simulink model "AXI_QPSK_Rx"  (R2017b)
settings: Solver=VariableStepAuto  StartTime=0.0  StopTime=2500/Rb  RelTol=1e-3
PreLoadFcn:
  | design_filters_rx;      % run script to generate filter designs.
  | 
  | Rb = 1000;   % 1kbit / s
  | 
  | Rsym = Rb/2;   % 2 bits per symbol
  | 
  | Rsymbol = Rb/2;
  | 
  | OSR = 32;
  | 
  | f_error = 120;
  | 
  | fc = 100e3;
values from neighbouring files (symbols this model uses):
  CIC_fine_Rx = 2^(-(CIC_right_shift_i-CIC_shift_Rx))    [design_filters_rx.m]
  fCIC = fCICcomp * R_CIC    (= 25600000)    [design_filters_rx.m]
  R_CIC = 3200    [design_filters_rx.m]
  R_CICcomp = 2    [design_filters_rx.m]
  R_HB = 2    [design_filters_rx.m]
  R_RRC = 4    [design_filters_rx.m]
undefined symbols (not defined in the file or in its folder): AXI4, designMultirateFIR, Lite
libraries: xbsIndex_r4 x539, dspmlti4 x12, dsparch4 x2, dspsrcs4 x2, commrandsrc2 x1, commdigbbndpm3 x1
(part 1 of 5)
CloseFcn:
  | clear
settings Model: Creator=nas07122  LastModifiedBy=jng
settings CodeAppCC: StateflowObjectComments=on

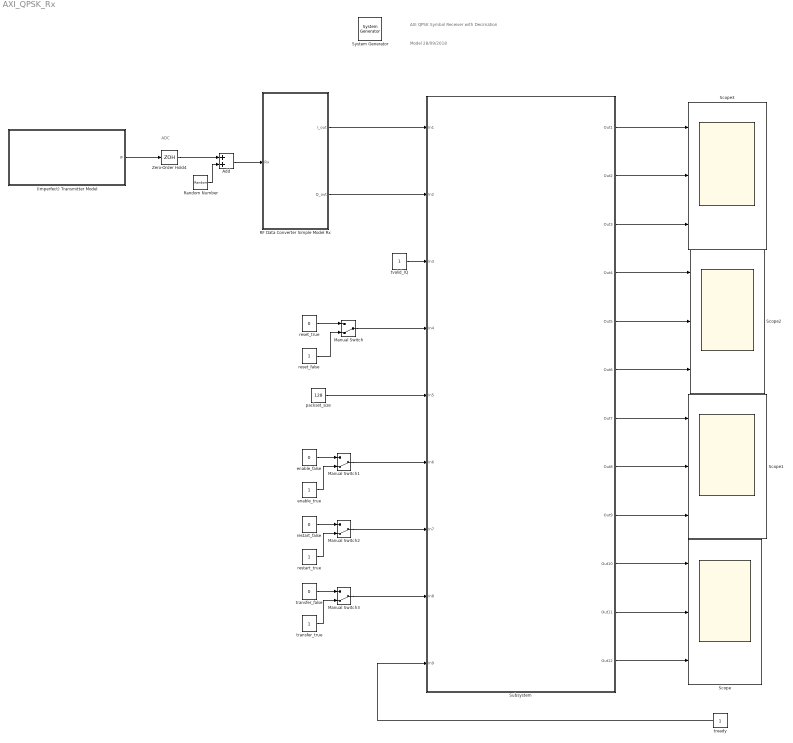
== system AXI_QPSK_Rx ==
  note: ADC
  note: AXI QPSK Symbol Receiver with Decimation
  note: Model 28/09/2018
  " System Generator" : xbsIndex_r4/ System Generator  Tag=genX  xilinxfamily=zynquplusRFSOC  part=xczu28dr  speed=-2-e  package=ffvg1517  synthesis_tool=Vivado  clock_wrapper=Clock Enables  directory=../../iprepo/zcu111/rx  proj_type=Vivado  Synth_file=Vivado Synthesis Defaults  Impl_file=Vivado Implementation Defaults  testbench=off  simulink_period=1/(0.5*Rb*R_RRC*R_HB*R_CICcomp*R_CIC)  sysclk_period=10  dcm_input_clock_period=10  incr_netlist=off  trim_vbits=Everywhere in SubSystem  dbl_ovrd=According to Block Masks  core_generation=According to Block Masks  run_coregen=off  deprecated_control=off  eval_field=0  block_type=sysgen
  (Imperfect) Transmitter Model : Subsystem  mask(Model of a QPSK Transmitter with Timing and Frequency Offsets){T_error=5, F_error=f_error, fc=fc}
      mask prompts: T_error "Timing Error (ppm)"; F_error "Frequency Error (Hz)"; fc "IF Carrier Frequency (Hz)"
      mask help:
      | Enter the timing and frequency offsets that apply to the received signal.
      |
      | Both of these can be negative or positive values. Negative means that the timing / frequency of the transmitter is lower than expected.
      mask init:
      | T_Offset = 1+(T_error/1e6);
      | F_Offset = F_error;
  Add : Sum
  Manual Switch{,1..3} (4 alike) : ManualSwitch  CurrentSetting=0
  RF Data Converter Simple Model Rx : Subsystem
  Random Number : RandomNumber  Variance=0.05  SampleTime=1/(0.5*R_RRC*R_HB*R_CICcomp*R_CIC*8*Rb)
  Scope{,1..3} (4 alike) : Scope  NumInputPorts=3
  Subsystem : Subsystem
  Zero-Order Hold4 : ZeroOrderHold  SampleTime=1/(0.5*R_RRC*R_HB*R_CICcomp*R_CIC*8*Rb)
  enable_false : Constant  Value=0  VectorParams1D=off  OutDataTypeStr=boolean  SampleTime=-1
  enable_true : Constant  VectorParams1D=off  OutDataTypeStr=boolean  SampleTime=-1
  packset_size : Constant  Value=128  SampleTime=-1
  reset_false : Constant  VectorParams1D=off  OutDataTypeStr=boolean  SampleTime=-1
  reset_true : Constant  Value=0  VectorParams1D=off  OutDataTypeStr=boolean  SampleTime=-1
  restart_false : Constant  Value=0  VectorParams1D=off  OutDataTypeStr=boolean  SampleTime=-1
  restart_true : Constant  VectorParams1D=off  OutDataTypeStr=boolean  SampleTime=-1
  transfer_false : Constant  Value=0  VectorParams1D=off  OutDataTypeStr=boolean  SampleTime=-1
  transfer_true : Constant  VectorParams1D=off  OutDataTypeStr=boolean  SampleTime=-1
  tready : Constant  SampleTime=-1
  tvalid_IQ : Constant  VectorParams1D=off  OutDataTypeStr=boolean  SampleTime=-1
  wires:
  Add/1 -> RF Data Converter Simple Model Rx/1(Rx)
  Zero-Order Hold4/1 -> Add/1
  Random Number/1 -> Add/2
  (Imperfect) Transmitter Model/1(IF) -> Zero-Order Hold4/1
  enable_true/1 -> Manual Switch1/2
  transfer_false/1 -> Manual Switch3/1
  reset_true/1 -> Manual Switch/1
  transfer_true/1 -> Manual Switch3/2
  restart_false/1 -> Manual Switch2/1
  enable_false/1 -> Manual Switch1/1
  restart_true/1 -> Manual Switch2/2
  reset_false/1 -> Manual Switch/2
  RF Data Converter Simple Model Rx/1(I_out) -> Subsystem/1(In1)
  RF Data Converter Simple Model Rx/2(Q_out) -> Subsystem/2(In2)
  tvalid_IQ/1 -> Subsystem/3(In3)
  Manual Switch/1 -> Subsystem/4(In4)
  packset_size/1 -> Subsystem/5(In5)
  Manual Switch1/1 -> Subsystem/6(In6)
  Manual Switch2/1 -> Subsystem/7(In7)
  Manual Switch3/1 -> Subsystem/8(In8)
  tready/1 -> Subsystem/9(In9)
  Subsystem/1(Out1) -> Scope3/1
  Subsystem/2(Out2) -> Scope3/2
  Subsystem/3(Out3) -> Scope3/3
  Subsystem/4(Out4) -> Scope2/1
  Subsystem/5(Out5) -> Scope2/2
  Subsystem/6(Out6) -> Scope2/3
  Subsystem/7(Out7) -> Scope1/1
  Subsystem/8(Out8) -> Scope1/2
  Subsystem/9(Out9) -> Scope1/3
  Subsystem/10(Out10) -> Scope/1
  Subsystem/11(Out11) -> Scope/2
  Subsystem/12(Out12) -> Scope/3

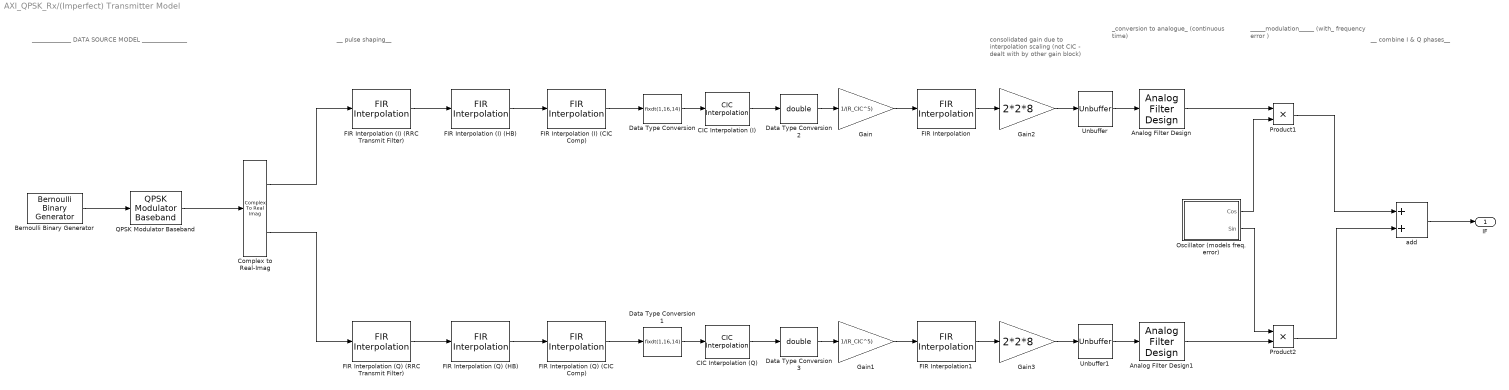
== system AXI_QPSK_Rx/(Imperfect) Transmitter Model ==
  note: consolidated gain
      | due to interpolation scaling
      | (not CIC - dealt with by other
      | gain block)
  note: _____________ DATA SOURCE MODEL _______________
  note: _conversion to analogue_
      | (continuous time)
  note: __ pulse shaping__
  note: _____modulation_____
      | (with_ frequency error )
  note: __ combine I & Q phases__
  Analog Filter Design : dsparch4/Analog Filter Design  method=Butterworth  filttype=Lowpass  N=8  Wlo=2*pi*Rsymbol*T_Offset  Whi=80  Rp=2  Rs=40
  Analog Filter Design1 : dsparch4/Analog Filter Design  method=Butterworth  filttype=Lowpass  N=8  Wlo=2*pi*Rsymbol*T_Offset  Whi=80  Rp=2  Rs=40
  Bernoulli Binary Generator : commrandsrc2/Bernoulli Binary Generator  P=0.5  seed=61  Ts=1/(T_Offset*Rb)  frameBased=on  sampPerFrame=2  orient=off  outDataType=double
  CIC Interpolation (I) : dspmlti4/CIC Interpolation  filtFrom=Dialog  filtobj=CICINTERP  ftype=Interpolator  R=R_CIC  M=1  N=5  filterInternals=Full precision  BPS=[16 16 16 16]  FLPS=0  outputWordLength=32  outputFracLength=0  launchFVT=off  framing=Enforce single-rate processing  InputProcessing=Columns as channels (frame based)  OutputFrames=off
      settings: SourceProductName=DSP System Toolbox  SourceProductBaseCode=DS
  CIC Interpolation (Q) : dspmlti4/CIC Interpolation  filtFrom=Dialog  filtobj=CICINTERP  ftype=Interpolator  R=R_CIC  M=1  N=5  filterInternals=Full precision  BPS=[16 16 16 16]  FLPS=0  outputWordLength=32  outputFracLength=0  launchFVT=off  framing=Enforce single-rate processing  InputProcessing=Columns as channels (frame based)  OutputFrames=off
      settings: SourceProductName=DSP System Toolbox  SourceProductBaseCode=DS
  Complex to Real-Imag : ComplexToRealImag
  Data Type Conversion : DataTypeConversion  OutDataTypeStr=fixdt(1,16,14)
  Data Type Conversion1 : DataTypeConversion  OutDataTypeStr=fixdt(1,16,14)
  Data Type Conversion2 : DataTypeConversion  OutDataTypeStr=double
  Data Type Conversion3 : DataTypeConversion  OutDataTypeStr=double
  FIR Interpolation : dspmlti4/FIR Interpolation  FilterSource=Auto  h=designMultirateFIR(3,1)  L=8  FilterObject=FINTERP  InputProcessing=Columns as channels (frame based)  framing=Allow multirate processing  outputBufInitCond=0  roundingMode=Floor  overflowMode=off  firstCoeffDataTypeStr=Inherit: Same word length as input  firstCoeffMin=[]  firstCoeffMax=[]  firstCoeffLastDataTypeStr=Inherit: Same word length as input  outputDataTypeStr=Inherit: Same as accumulator  outputMin=[]  outputMax=[]  outputLastDataTypeStr=Inherit: Same as accumulator
      settings: SourceProductName=DSP System Toolbox
  FIR Interpolation1 : dspmlti4/FIR Interpolation  FilterSource=Auto  h=designMultirateFIR(3,1)  L=8  FilterObject=FINTERP  InputProcessing=Columns as channels (frame based)  framing=Allow multirate processing  outputBufInitCond=0  roundingMode=Floor  overflowMode=off  firstCoeffDataTypeStr=Inherit: Same word length as input  firstCoeffMin=[]  firstCoeffMax=[]  firstCoeffLastDataTypeStr=Inherit: Same word length as input  outputDataTypeStr=Inherit: Same as accumulator  outputMin=[]  outputMax=[]  outputLastDataTypeStr=Inherit: Same as accumulator
      settings: SourceProductName=DSP System Toolbox
  FIR Interpolation (I) (CIC Comp) : dspmlti4/FIR Interpolation  FilterSource=Dialog parameters  h=WComp.Numerator  L=R_CICcomp  FilterObject=FINTERP  InputProcessing=Columns as channels (frame based)  framing=Allow multirate processing  outputBufInitCond=0  roundingMode=Floor  overflowMode=off  firstCoeffDataTypeStr=Inherit: Same word length as input  firstCoeffMin=[]  firstCoeffMax=[]  firstCoeffLastDataTypeStr=Inherit: Same word length as input  outputDataTypeStr=Inherit: Same as accumulator  outputMin=[]  outputMax=[]  outputLastDataTypeStr=Inherit: Same as accumulator
      settings: SourceProductName=DSP System Toolbox
  FIR Interpolation (I) (HB) : dspmlti4/FIR Interpolation  FilterSource=Dialog parameters  h=HB.Numerator  L=2  FilterObject=FINTERP  InputProcessing=Columns as channels (frame based)  framing=Allow multirate processing  outputBufInitCond=0  roundingMode=Floor  overflowMode=off  firstCoeffDataTypeStr=Inherit: Same word length as input  firstCoeffMin=[]  firstCoeffMax=[]  firstCoeffLastDataTypeStr=Inherit: Same word length as input  outputDataTypeStr=Inherit: Same as accumulator  outputMin=[]  outputMax=[]  outputLastDataTypeStr=Inherit: Same as accumulator
      settings: SourceProductName=DSP System Toolbox
  FIR Interpolation (I) (RRC Transmit Filter) : dspmlti4/FIR Interpolation  FilterSource=Dialog parameters  h=WRRC.Numerator  L=R_RRC  FilterObject=FINTERP  InputProcessing=Columns as channels (frame based)  framing=Allow multirate processing  outputBufInitCond=0  roundingMode=Floor  overflowMode=off  firstCoeffDataTypeStr=Inherit: Same word length as input  firstCoeffMin=[]  firstCoeffMax=[]  firstCoeffLastDataTypeStr=Inherit: Same word length as input  outputDataTypeStr=Inherit: Same as accumulator  outputMin=[]  outputMax=[]  outputLastDataTypeStr=Inherit: Same as accumulator
      settings: SourceProductName=DSP System Toolbox
  FIR Interpolation (Q) (CIC Comp) : dspmlti4/FIR Interpolation  FilterSource=Dialog parameters  h=WComp.Numerator  L=R_CICcomp  FilterObject=FINTERP  InputProcessing=Columns as channels (frame based)  framing=Allow multirate processing  outputBufInitCond=0  roundingMode=Floor  overflowMode=off  firstCoeffDataTypeStr=Inherit: Same word length as input  firstCoeffMin=[]  firstCoeffMax=[]  firstCoeffLastDataTypeStr=Inherit: Same word length as input  outputDataTypeStr=Inherit: Same as accumulator  outputMin=[]  outputMax=[]  outputLastDataTypeStr=Inherit: Same as accumulator
      settings: SourceProductName=DSP System Toolbox
  FIR Interpolation (Q) (HB) : dspmlti4/FIR Interpolation  FilterSource=Dialog parameters  h=HB.Numerator  L=2  FilterObject=FINTERP  InputProcessing=Columns as channels (frame based)  framing=Allow multirate processing  outputBufInitCond=0  roundingMode=Floor  overflowMode=off  firstCoeffDataTypeStr=Inherit: Same word length as input  firstCoeffMin=[]  firstCoeffMax=[]  firstCoeffLastDataTypeStr=Inherit: Same word length as input  outputDataTypeStr=Inherit: Same as accumulator  outputMin=[]  outputMax=[]  outputLastDataTypeStr=Inherit: Same as accumulator
      settings: SourceProductName=DSP System Toolbox
  FIR Interpolation (Q) (RRC Transmit Filter) : dspmlti4/FIR Interpolation  FilterSource=Dialog parameters  h=WRRC.Numerator  L=R_RRC  FilterObject=FINTERP  InputProcessing=Columns as channels (frame based)  framing=Allow multirate processing  outputBufInitCond=0  roundingMode=Floor  overflowMode=off  firstCoeffDataTypeStr=Inherit: Same word length as input  firstCoeffMin=[]  firstCoeffMax=[]  firstCoeffLastDataTypeStr=Inherit: Same word length as input  outputDataTypeStr=Inherit: Same as accumulator  outputMin=[]  outputMax=[]  outputLastDataTypeStr=Inherit: Same as accumulator
      settings: SourceProductName=DSP System Toolbox
  Gain : Gain  Gain=1/(R_CIC^5)
  Gain1 : Gain  Gain=1/(R_CIC^5)
  Gain2 : Gain  Gain=2*2*8
  Gain3 : Gain  Gain=2*2*8
  Oscillator (models freq. error) : Subsystem
  Product1 : Product
  Product2 : Product
  QPSK Modulator Baseband : commdigbbndpm3/QPSK Modulator Baseband  InType=Bit  Enc=Gray  Ph=pi/4  outDtype=double  outWordLen=16  outUDDataType=sfix(16)  outFracLenMode=Best precision  outFracLen=15  outDataTypeStr=double  outLastDataTypeStr=double
  Unbuffer : Unbuffer
  Unbuffer1 : Unbuffer
  add : Sum
  IF : Outport
  wires:
  FIR Interpolation (Q) (RRC Transmit Filter)/1 -> FIR Interpolation (Q) (HB)/1
  Complex to Real-Imag/2 -> FIR Interpolation (Q) (RRC Transmit Filter)/1
  Complex to Real-Imag/1 -> FIR Interpolation (I) (RRC Transmit Filter)/1
  Bernoulli Binary Generator/1 -> QPSK Modulator Baseband/1
  FIR Interpolation (I) (RRC Transmit Filter)/1 -> FIR Interpolation (I) (HB)/1
  Product1/1 -> add/1
  Analog Filter Design/1 -> Product1/1
  Analog Filter Design1/1 -> Product2/2
  Product2/1 -> add/2
  add/1 -> IF/1
  Oscillator (models freq. error)/1(Cos) -> Product1/2
  Oscillator (models freq. error)/2(Sin) -> Product2/1
  QPSK Modulator Baseband/1 -> Complex to Real-Imag/1
  Unbuffer/1 -> Analog Filter Design/1
  Unbuffer1/1 -> Analog Filter Design1/1
  FIR Interpolation (I) (HB)/1 -> FIR Interpolation (I) (CIC Comp)/1
  FIR Interpolation (Q) (HB)/1 -> FIR Interpolation (Q) (CIC Comp)/1
  FIR Interpolation (I) (CIC Comp)/1 -> Data Type Conversion/1
  FIR Interpolation (Q) (CIC Comp)/1 -> Data Type Conversion1/1
  CIC Interpolation (I)/1 -> Data Type Conversion2/1
  CIC Interpolation (Q)/1 -> Data Type Conversion3/1
  FIR Interpolation/1 -> Gain2/1
  FIR Interpolation1/1 -> Gain3/1
  Data Type Conversion/1 -> CIC Interpolation (I)/1
  Data Type Conversion1/1 -> CIC Interpolation (Q)/1
  Data Type Conversion2/1 -> Gain/1
  Data Type Conversion3/1 -> Gain1/1
  Gain/1 -> FIR Interpolation/1
  Gain1/1 -> FIR Interpolation1/1
  Gain2/1 -> Unbuffer/1
  Gain3/1 -> Unbuffer1/1

== system AXI_QPSK_Rx/RF Data Converter Simple Model Rx ==
  Rx : Inport
  Cosine Wave : dspsrcs4/Sine Wave  Amplitude=1  Frequency=fc  Phase=pi/2  SampleMode=Discrete  OutComplex=Real  CompMethod=Trigonometric fcn  TableSize=Speed  SampleTime=1/(0.5*R_RRC*R_HB*R_CICcomp*R_CIC*8*Rb)  SamplesPerFrame=1  ResetState=Restart at time zero  OutputFrames=off  dataType=double  wordLen=16  udDataType=sfix(16)  fracBitsMode=Best precision  numFracBits=15  OutDataTypeStr=double  LastOutDataTypeStr=double
  FIR Decimation : dspmlti4/FIR Decimation  FilterSource=Auto  h=designMultirateFIR(1,2)  D=8  filtStruct=Direct form  FilterObject=FDECIM  framing=Enforce single-rate processing  inputOffset=0  outputBufInitCond=0  roundingMode=Floor  overflowMode=off  firstCoeffDataTypeStr=Inherit: Same word length as input  firstCoeffMin=[]  firstCoeffMax=[]  firstCoeffLastDataTypeStr=Inherit: Same word length as input  outputDataTypeStr=Inherit: Same as accumulator  outputMin=[]  outputMax=[]  outputLastDataTypeStr=Inherit: Same as accumulator
  FIR Decimation1 : dspmlti4/FIR Decimation  FilterSource=Auto  h=designMultirateFIR(1,2)  D=8  filtStruct=Direct form  FilterObject=FDECIM  framing=Enforce single-rate processing  inputOffset=0  outputBufInitCond=0  roundingMode=Floor  overflowMode=off  firstCoeffDataTypeStr=Inherit: Same word length as input  firstCoeffMin=[]  firstCoeffMax=[]  firstCoeffLastDataTypeStr=Inherit: Same word length as input  outputDataTypeStr=Inherit: Same as accumulator  outputMin=[]  outputMax=[]  outputLastDataTypeStr=Inherit: Same as accumulator
  Product : Product
  Product1 : Product
  Sine Wave : dspsrcs4/Sine Wave  Amplitude=1  Frequency=fc  Phase=pi  SampleMode=Discrete  OutComplex=Real  CompMethod=Trigonometric fcn  TableSize=Speed  SampleTime=1/(0.5*R_RRC*R_HB*R_CICcomp*R_CIC*8*Rb)  SamplesPerFrame=1  ResetState=Restart at time zero  OutputFrames=off  dataType=double  wordLen=16  udDataType=sfix(16)  fracBitsMode=Best precision  numFracBits=15  OutDataTypeStr=double  LastOutDataTypeStr=double
  I_out : Outport
  Q_out : Outport  Port=2
  wires:
  FIR Decimation/1 -> I_out/1
  Rx/1 -> Product1/2, Product/1
  Cosine Wave/1 -> Product/2
  Product/1 -> FIR Decimation/1
  Sine Wave/1 -> Product1/1
  Product1/1 -> FIR Decimation1/1
  FIR Decimation1/1 -> Q_out/1

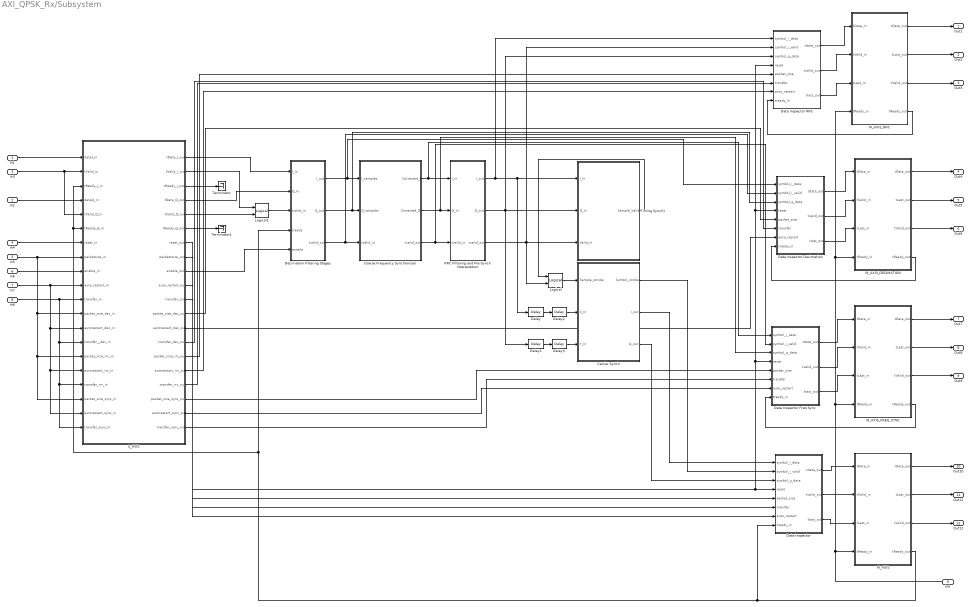
== system AXI_QPSK_Rx/Subsystem ==
  In1 : Inport
  In2 : Inport  Port=2
  In3 : Inport  Port=3
  In4 : Inport  Port=4
  In5 : Inport  Port=5
  In6 : Inport  Port=6
  In7 : Inport  Port=7
  In8 : Inport  Port=8
  In9 : Inport  Port=9
  Carrier Synch : Subsystem  mask(Symbol Timing Synchroniser){Rsymbol=Rsymbol}
      mask prompts: Rsymbol "Symbol rate (Hz)"
      mask init:
      | d = 0.707;                  % damping ratio 
      | 
      | % *** CARRIER synch loop *** (note this operates at symbol rate)
      | 
      | T = 1/Rsymbol;               % sample period
      | Kp = 1;                      % phase detector S-curve is linear
      | Bn = 0.04*Rsymbol;           % bandwidth in Hz
      | Ko = 1;                      % gain of NCO 
      | 
      | % calculate the loop filter coefficients for the carrier synch loop
      | K1 = (4*d*Bn*T)/(Ko*Kp*(d+1/(4*d)));
      | K2 = (4*(Bn*T)^2)/(Ko*Kp*(d+1/4*d)^2);
  Coarse Frequency Synchroniser : Subsystem  mask(Coarse Frequency Synchronisation (QPSK)){f_coarse=(0.5*R_RRC*R_HB*Rb), Nfft=512}
      mask prompts: f_coarse "Sampling frequency"; Nfft "FFT size (must be power of 2)"
      mask help: This coarse synchronisation block raises the received signal to the power of M = 4 (for QPSK, i.e. the modulation order) and finds the peak in the resulting spectrum, to identify the frequency offset from baseband. A complex exponential at the identified frequency is then generated and used to perform a frequency correction on the received signal.
      mask init:
      | M = 4;      % for QPSK
      | 
      | % set FFT block to size specified in mask.
      | set_param([gcb,'/FFT'],'transform_length',num2str(Nfft));      
      | 
      | % generate lookup table for frequency correction term
      | fcorr_lookup = zeros(1,Nfft);
      | 
      | n = (0:Nfft-1);
      | fcorr_lookup(1:Nfft/2) = - (n(1:Nfft/2) * (f_coarse/(4*Nfft)));
      | fcorr_lookup((Nfft/2)+1:end) = - ((n((Nfft/2)+1:end) - Nfft) *  (f_coarse/(4*Nfft)));
  Data Inspector : Subsystem
  Data Inspector Decimation : Subsystem
  Data Inspector Freq Sync : Subsystem
  Data Inspector RRC : Subsystem
  Decimation Filtering Stages : Subsystem
  Delay : xbsIndex_r4/Delay  rst=off  infoeditControl=Selection of Reset will increase slice count due to use of real FFs and instead of SRLs  en=off  latency=OSR/2  reg_retiming=off  dbl_ovrd=off  block_type=delay
  Delay1 : xbsIndex_r4/Delay  rst=off  infoeditControl=Selection of Reset will increase slice count due to use of real FFs and instead of SRLs  en=off  latency=OSR/2  reg_retiming=off  dbl_ovrd=off  block_type=delay
  Delay2 : xbsIndex_r4/Delay  rst=off  infoeditControl=Selection of Reset will increase slice count due to use of real FFs and instead of SRLs  en=off  latency=1  reg_retiming=off  dbl_ovrd=off  block_type=delay
  Delay3 : xbsIndex_r4/Delay  rst=off  infoeditControl=Selection of Reset will increase slice count due to use of real FFs and instead of SRLs  en=off  latency=1  reg_retiming=off  dbl_ovrd=off  block_type=delay
  Logical : xbsIndex_r4/Logical  logical_function=AND  inputs=2  en=off  latency=0  precision=Full  arith_type=Unsigned  n_bits=16  bin_pt=0  align_bp=on  dbl_ovrd=off  block_type=logical
  Logical1 : xbsIndex_r4/Logical  logical_function=AND  inputs=2  en=off  latency=0  precision=Full  arith_type=Unsigned  n_bits=16  bin_pt=0  align_bp=on  dbl_ovrd=off  block_type=logical
  M_AXIS : Subsystem
  M_AXIS_DECIMATION : Subsystem
  M_AXIS_FREQ_SYNC : Subsystem
  M_AXIS_RRC : Subsystem
  "RRC Filtering and Pre-Synch Interpolation " : Subsystem
  S_AXIS : Subsystem
  Terminator : Terminator
  Terminator1 : Terminator
  Timing Synch1 : Subsystem  mask(Symbol Timing Synchroniser){Rsymbol=Rsymbol}
      mask prompts: Rsymbol "Symbol rate (Hz)"
      mask init:
      | % *** SYMBOL TIMING synch loop ***
      | 
      | d = 0.707;                  % damping ratio 
      | Ts = 1/Rsymbol;             % symbol period
      | Ks = 3.24;                  % phase detector coefficient
      | BnS = 0.08*Rsymbol;         % bandwidth in Hz
      | Kn   = 1;                   % gain of numerically controlled clock
      | 
      | % calculate loop filter coefficients
      | Ka = (4*d*BnS*Ts)/(Kn*Ks*(d+1/(4*d)));
      | Kb = (4*(BnS*Ts)^2)/(Kn*Ks*(d+1/4*d)^2);
  Out1 : Outport
  Out2 : Outport  Port=2
  Out3 : Outport  Port=3
  Out4 : Outport  Port=4
  Out5 : Outport  Port=5
  Out6 : Outport  Port=6
  Out7 : Outport  Port=7
  Out8 : Outport  Port=8
  Out9 : Outport  Port=9
  Out10 : Outport  Port=10
  Out11 : Outport  Port=11
  Out12 : Outport  Port=12
  wires:
  Coarse Frequency Synchroniser/1(Corrected_I) -> Data Inspector Freq Sync/1(symbol_i_data), "RRC Filtering and Pre-Synch Interpolation "/1(I_in)
  In2/1 -> S_AXIS/4(dataQ_in)
  M_AXIS_FREQ_SYNC/1(tData_out) -> Out7/1
  Data Inspector Freq Sync/2(tvalid_out) -> M_AXIS_FREQ_SYNC/2(tValid_in)
  In5/1 -> S_AXIS/8(packetsize_in), S_AXIS/12(packet_size_dec_in), S_AXIS/15(packet_size_rrc_in), S_AXIS/18(packet_size_sync_in)
  S_AXIS/16(autorestart_rrc_out) -> Data Inspector RRC/7(auto_restart)
  S_AXIS/19(autorestart_sync_out) -> Data Inspector Freq Sync/7(auto_restart)
  S_AXIS/10(auto_restart_out) -> Data Inspector/7(auto_restart)
  S_AXIS/13(autorestart_dec_out) -> Data Inspector Decimation/7(auto_restart)
  S_AXIS/1(tData_I_out) -> Decimation Filtering Stages/1(I_In)
  In9/1 -> M_AXIS/4(tReady_in), M_AXIS_FREQ_SYNC/4(tReady_in), M_AXIS_DECIMATION/4(tReady_in), M_AXIS_RRC/4(tReady_in)
  S_AXIS/6(tReady_Q_out) -> Terminator1/1
  Data Inspector/2(tvalid_out) -> M_AXIS/2(tValid_in)
  M_AXIS_DECIMATION/4(tReady_out) -> Data Inspector Decimation/8(tready_in)
  In6/1 -> S_AXIS/9(enable_in)
  Timing Synch1/1(Sample_Valid) -> Logical/1
  "RRC Filtering and Pre-Synch Interpolation "/3(tvalid_out) -> Data Inspector RRC/2(symbol_i_valid), Timing Synch1/3(Valid_in), Logical/2
  M_AXIS_DECIMATION/2(tLast_out) -> Out5/1
  Delay/1 -> Delay2/1
  Delay1/1 -> Delay3/1
  Logical1/1 -> Decimation Filtering Stages/3(tvalid_in)
  Logical/1 -> Carrier Synch/1(Sample_strobe)
  M_AXIS_FREQ_SYNC/2(tLast_out) -> Out8/1
  Carrier Synch/1(Symbol_strobe) -> Data Inspector/2(symbol_i_valid)
  S_AXIS/2(tValid_I_out) -> Logical1/1
  M_AXIS_RRC/3(tValid_out) -> Out3/1
  M_AXIS_FREQ_SYNC/4(tReady_out) -> Data Inspector Freq Sync/8(tready_in)
  S_AXIS/5(tValid_Q_out) -> Logical1/2
  Carrier Synch/3(Q_out) -> Data Inspector/3(symbol_q_data)
  Decimation Filtering Stages/2(Q_out) -> Data Inspector Decimation/3(symbol_q_data), Coarse Frequency Synchroniser/2(Q_samples)
  In8/1 -> S_AXIS/11(transfer_in), S_AXIS/14(transfer__dec_in), S_AXIS/17(transfer_rrc_in), S_AXIS/20(transfer_sync_in)
  Data Inspector Decimation/3(tlast_out) -> M_AXIS_DECIMATION/3(tLast_in)
  Data Inspector/3(tlast_out) -> M_AXIS/3(tLast_in)
  S_AXIS/4(tData_Q_out) -> Decimation Filtering Stages/2(Q_In)
  Data Inspector RRC/2(tvalid_out) -> M_AXIS_RRC/2(tValid_in)
  S_AXIS/18(packet_size_sync_out) -> Data Inspector Freq Sync/5(packet_size)
  M_AXIS_DECIMATION/3(tValid_out) -> Out6/1
  Data Inspector RRC/1(tdata_out) -> M_AXIS_RRC/1(tData_in)
  In3/1 -> S_AXIS/5(tValid_Q_in), S_AXIS/2(tValid_in)
  Data Inspector Freq Sync/1(tdata_out) -> M_AXIS_FREQ_SYNC/1(tData_in)
  Coarse Frequency Synchroniser/3(tvalid_out) -> Data Inspector Freq Sync/2(symbol_i_valid), "RRC Filtering and Pre-Synch Interpolation "/3(tvalid_in)
  Data Inspector RRC/3(tlast_out) -> M_AXIS_RRC/3(tLast_in)
  Data Inspector Decimation/2(tvalid_out) -> M_AXIS_DECIMATION/2(tValid_in)
  In7/1 -> S_AXIS/19(autorestart_sync_in), S_AXIS/16(autorestart_rrc_in), S_AXIS/13(autorestart_dec_in), S_AXIS/10(auto_restart_in)
  M_AXIS_RRC/4(tReady_out) -> Data Inspector RRC/8(tready_in)
  M_AXIS/3(tValid_out) -> Out12/1
  Data Inspector/1(tdata_out) -> M_AXIS/1(tData_in)
  S_AXIS/8(packsetsize_out) -> Data Inspector/5(packet_size)
  S_AXIS/14(transfer_dec_out) -> Data Inspector Decimation/6(transfer)
  Data Inspector Freq Sync/3(tlast_out) -> M_AXIS_FREQ_SYNC/3(tLast_in)
  S_AXIS/11(transfer_out) -> Data Inspector/6(transfer)
  Delay2/1 -> Carrier Synch/2(X_In)
  Data Inspector Decimation/1(tdata_out) -> M_AXIS_DECIMATION/1(tData_in)
  S_AXIS/15(packet_size_rrc_out) -> Data Inspector RRC/5(packet_size)
  Delay3/1 -> Carrier Synch/3(Y_In)
  M_AXIS_DECIMATION/1(tData_out) -> Out4/1
  S_AXIS/3(tReady_I_out) -> Terminator/1
  M_AXIS/4(tReady_out) -> S_AXIS/3(tReady_I_in), S_AXIS/6(tReady_Q_in), Decimation Filtering Stages/4(tready), Data Inspector/8(tready_in)
  S_AXIS/9(enable_out) -> Decimation Filtering Stages/5(enable)
  In4/1 -> S_AXIS/7(reset_in)
  Carrier Synch/2(I_out) -> Data Inspector/1(symbol_i_data)
  "RRC Filtering and Pre-Synch Interpolation "/2(Q_out) -> Data Inspector RRC/3(symbol_q_data), Timing Synch1/2(Q_In), Delay1/1
  S_AXIS/7(reset_out) -> Data Inspector Decimation/4(reset), Data Inspector RRC/4(reset), Data Inspector Freq Sync/4(reset), Data Inspector/4(reset)
  S_AXIS/17(transfer_rrc_out) -> Data Inspector RRC/6(transfer)
  M_AXIS_RRC/1(tData_out) -> Out1/1
  M_AXIS_RRC/2(tLast_out) -> Out2/1
  M_AXIS_FREQ_SYNC/3(tValid_out) -> Out9/1
  M_AXIS/1(tData_out) -> Out10/1
  M_AXIS/2(tLast_out) -> Out11/1
  In1/1 -> S_AXIS/1(dataI_in)
  Decimation Filtering Stages/3(tvalid_out) -> Data Inspector Decimation/2(symbol_i_valid), Coarse Frequency Synchroniser/3(tvalid_in)
  S_AXIS/20(transfer_sync_out) -> Data Inspector Freq Sync/6(transfer)
  "RRC Filtering and Pre-Synch Interpolation "/1(I_out) -> Data Inspector RRC/1(symbol_i_data), Timing Synch1/1(I_In), Delay/1
  Coarse Frequency Synchroniser/2(Corrected_Q) -> Data Inspector Freq Sync/3(symbol_q_data), "RRC Filtering and Pre-Synch Interpolation "/2(Q_in)
  S_AXIS/12(packet_size_dec_out) -> Data Inspector Decimation/5(packet_size)
  Decimation Filtering Stages/1(I_out) -> Data Inspector Decimation/1(symbol_i_data), Coarse Frequency Synchroniser/1(I_samples)

== system AXI_QPSK_Rx/(Imperfect) Transmitter Model/Oscillator (models freq. error) ==
  Cosine Wave : Sin  Frequency=2*pi*(fc-F_Offset)  Phase=pi/2  SampleTime=0
  Sine Wave : Sin  Frequency=2*pi*(fc-F_Offset)  SampleTime=0
  Cos : Outport
  Sin : Outport  Port=2
  wires:
  Sine Wave/1 -> Sin/1
  Cosine Wave/1 -> Cos/1

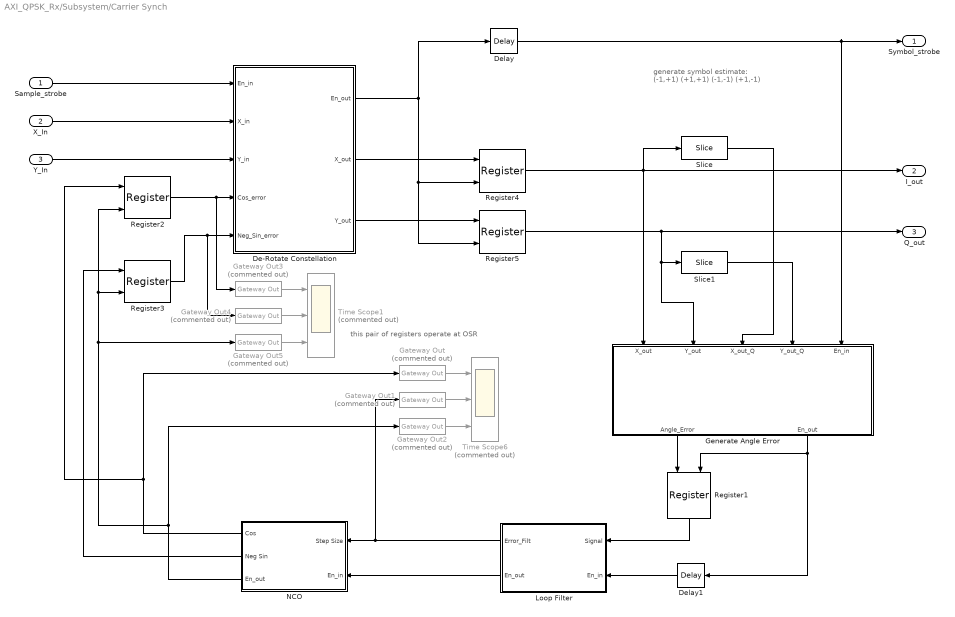
== system AXI_QPSK_Rx/Subsystem/Carrier Synch ==
  note: this pair of registers operate at OSR
  note: generate symbol estimate:
      |
      |           (-1,+1)                 (+1,+1)
      |
      |
      |           (-1,-1)                  (+1,-1)
  Sample_strobe : Inport
  X_In : Inport  Port=2
  Y_In : Inport  Port=3
  De-Rotate Constellation : Subsystem
  Delay : xbsIndex_r4/Delay  rst=off  infoeditControl=Selection of Reset will increase slice count due to use of real FFs and instead of SRLs  en=off  latency=1  reg_retiming=off  dbl_ovrd=off  block_type=delay
  Delay1 : xbsIndex_r4/Delay  rst=off  infoeditControl=Selection of Reset will increase slice count due to use of real FFs and instead of SRLs  en=off  latency=1  reg_retiming=off  dbl_ovrd=off  block_type=delay
  Gateway Out{,1..5} (6 alike) : xbsIndex_r4/Gateway Out  Commented=on  inherit_from_input=off  hdl_port=on  rows=1  columns=1  UseAsDAC=off  DACChannel='1'  interface=None  automatic_assignment=on  address_offset=hex2dec('00')  intf_name=''  intf_description=''  timing_constraint=None  locs_specified=off  LOCs={}  io_standard={}  block_type=gatewayout
  Generate Angle Error : Subsystem
  Loop Filter : Subsystem  mask(Loop Filter){K1=K1, K2=K2}
      mask prompts: K1 "Proportional gain (K1)"; K2 "Integral gain (K2)"
      mask help:
      | Filters the error signal generated within the Carrier Synchronisation Loop.
      |
      | Key parameters are the gain of the proportional and integral branches.
  NCO : Subsystem  mask(NCO){n=8, b=14}
      mask prompts: n "Number of integer_bits"; b "Number of fractional bits"
      mask help:
      | Numerically Controller Oscillator.
      |
      | Integrates the phase error and generates cosine and negative sign outputs.
      mask init:
      | k_n = ceil(log2((2^n)/(2*pi)))
      mask DialogControl Container3 Prompt: Accumulator
  Register1 : xbsIndex_r4/Register  init=0  rst=off  en=on  dbl_ovrd=off  block_type=register
  Register2 : xbsIndex_r4/Register  init=1  rst=off  en=on  dbl_ovrd=off  block_type=register
  Register3 : xbsIndex_r4/Register  init=0  rst=off  en=on  dbl_ovrd=off  block_type=register
  Register4 : xbsIndex_r4/Register  init=1  rst=off  en=on  dbl_ovrd=off  block_type=register
  Register5 : xbsIndex_r4/Register  init=1  rst=off  en=on  dbl_ovrd=off  block_type=register
  Slice : xbsIndex_r4/Slice  nbits=1  boolean_output=off  mode=Upper Bit Location + Width  bit1=0  base1=MSB of Input  bit0=0  base0=LSB of Input  dbl_ovrd=off  block_type=slice
  Slice1 : xbsIndex_r4/Slice  nbits=1  boolean_output=off  mode=Upper Bit Location + Width  bit1=0  base1=MSB of Input  bit0=0  base0=LSB of Input  dbl_ovrd=off  block_type=slice
  Time Scope1 : Scope  Commented=on  NumInputPorts=3
  Time Scope6 : Scope  Commented=on  NumInputPorts=3
  Symbol_strobe : Outport
  I_out : Outport  Port=2
  Q_out : Outport  Port=3
  wires:
  X_In/1 -> De-Rotate Constellation/2(X_in)
  Y_In/1 -> De-Rotate Constellation/3(Y_in)
  Register4/1 -> Slice/1, I_out/1, Generate Angle Error/1(X_out)
  Register5/1 -> Q_out/1, Generate Angle Error/2(Y_out), Slice1/1
  Slice/1 -> Generate Angle Error/3(X_out_Q)
  Slice1/1 -> Generate Angle Error/4(Y_out_Q)
  Register1/1 -> Loop Filter/1(Signal)
  Loop Filter/2(En_out) -> NCO/2(En_in)
  Loop Filter/1(Error_Filt) -> Gateway Out1/1, NCO/1(Step Size)
  Register2/1 -> Gateway Out3/1, De-Rotate Constellation/4(Cos_error)
  Register3/1 -> Gateway Out4/1, De-Rotate Constellation/5(Neg_Sin_error)
  NCO/1(Cos) -> Gateway Out/1, Register2/1
  NCO/2(Neg Sin) -> Register3/1
  NCO/3(En_out) -> Gateway Out2/1, Gateway Out5/1, Register2/2, Register3/2
  Sample_strobe/1 -> De-Rotate Constellation/1(En_in)
  De-Rotate Constellation/1(En_out) -> Delay/1, Register4/2, Register5/2
  Delay/1 -> Symbol_strobe/1, Generate Angle Error/5(En_in)
  Gateway Out/1 -> Time Scope6/1
  Gateway Out1/1 -> Time Scope6/2
  Gateway Out2/1 -> Time Scope6/3
  Generate Angle Error/1(Angle_Error) -> Register1/1
  Generate Angle Error/2(En_out) -> Delay1/1, Register1/2
  Delay1/1 -> Loop Filter/2(En_in)
  Gateway Out5/1 -> Time Scope1/3
  Gateway Out4/1 -> Time Scope1/2
  Gateway Out3/1 -> Time Scope1/1
  De-Rotate Constellation/2(X_out) -> Register4/1
  De-Rotate Constellation/3(Y_out) -> Register5/1

== system AXI_QPSK_Rx/Subsystem/Coarse Frequency Synchroniser ==
  note: Raise input to power of 4 (M = 4 for QPSK)
  note: FFT (generates Xk and index k)
  note: Process FFT Results to Determine
      | Required Frequency Correction
  note: NCO to Generate
      | Correction Signal
  note: Apply Correction
  I_samples : Inport
  Q_samples : Inport  Port=2
  tvalid_in : Inport  Port=3
  Constant2 : xbsIndex_r4/Constant  const=1  gui_display_data_type=Boolean  arith_type=Boolean  n_bits=9  bin_pt=0  preci_type=Single  exp_width=8  frac_width=24  explicit_period=on  period=1/f_coarse  equ=P=C  opselect=C  inp2=PCIN>>17  opr=+  inp1=P  carry=CIN  dbl_ovrd=off  block_type=constant
  Constant3 : xbsIndex_r4/Constant  const=1  gui_display_data_type=Fixed-point  arith_type=Unsigned  n_bits=1  bin_pt=0  preci_type=Single  exp_width=8  frac_width=24  explicit_period=on  period=1/f_coarse  equ=P=C  opselect=C  inp2=PCIN>>17  opr=+  inp1=P  carry=CIN  dbl_ovrd=off  block_type=constant
  Constant4 : xbsIndex_r4/Constant  const=1  gui_display_data_type=Boolean  arith_type=Boolean  n_bits=9  bin_pt=0  preci_type=Single  exp_width=8  frac_width=24  explicit_period=on  period=1/f_coarse  equ=P=C  opselect=C  inp2=PCIN>>17  opr=+  inp1=P  carry=CIN  dbl_ovrd=off  block_type=constant
  Convert : xbsIndex_r4/Convert  gui_display_data_type=Fixed-point  arith_type="Signed  (2's comp)"  n_bits=19  bin_pt=14  float_type=Single  exp_bits=8  fraction_bits=24  quantization=Truncate  overflow=Wrap  en=off  latency=0  pipeline=off  dbl_ovrd=off  block_type=convert
  Convert1 : xbsIndex_r4/Convert  gui_display_data_type=Fixed-point  arith_type="Signed  (2's comp)"  n_bits=19  bin_pt=14  float_type=Single  exp_bits=8  fraction_bits=24  quantization=Truncate  overflow=Wrap  en=off  latency=0  pipeline=off  dbl_ovrd=off  block_type=convert
  Convert2 : xbsIndex_r4/Convert  gui_display_data_type=Fixed-point  arith_type="Signed  (2's comp)"  n_bits=16  bin_pt=15  float_type=Single  exp_bits=8  fraction_bits=24  quantization=Truncate  overflow=Wrap  en=off  latency=0  pipeline=off  dbl_ovrd=off  block_type=convert
  Convert3 : xbsIndex_r4/Convert  gui_display_data_type=Fixed-point  arith_type="Signed  (2's comp)"  n_bits=16  bin_pt=15  float_type=Single  exp_bits=8  fraction_bits=24  quantization=Truncate  overflow=Wrap  en=off  latency=0  pipeline=off  dbl_ovrd=off  block_type=convert
  Convert4 : xbsIndex_r4/Convert  gui_display_data_type=Fixed-point  arith_type="Signed  (2's comp)"  n_bits=18  bin_pt=15  float_type=Single  exp_bits=8  fraction_bits=24  quantization=Truncate  overflow=Wrap  en=off  latency=0  pipeline=off  dbl_ovrd=off  block_type=convert
  Convert5 : xbsIndex_r4/Convert  gui_display_data_type=Fixed-point  arith_type="Signed  (2's comp)"  n_bits=18  bin_pt=15  float_type=Single  exp_bits=8  fraction_bits=24  quantization=Truncate  overflow=Wrap  en=off  latency=0  pipeline=off  dbl_ovrd=off  block_type=convert
  Delay : xbsIndex_r4/Delay  rst=off  infoeditControl=Selection of Reset will increase slice count due to use of real FFs and instead of SRLs  en=off  latency=6  reg_retiming=off  dbl_ovrd=off  block_type=delay
  Delay1 : xbsIndex_r4/Delay  rst=off  infoeditControl=Selection of Reset will increase slice count due to use of real FFs and instead of SRLs  en=off  latency=6  reg_retiming=off  dbl_ovrd=off  block_type=delay
  Delay2 : xbsIndex_r4/Delay  rst=off  infoeditControl=Selection of Reset will increase slice count due to use of real FFs and instead of SRLs  en=off  latency=6  reg_retiming=off  dbl_ovrd=off  block_type=delay
  Determine Frequency Correction Term : Subsystem
  FFT : xbsIndex_r4/Fast Fourier Transform 9.1   transform_length=512  target_clock_frequency=250  target_data_throughput=50  implementation_options=pipelined_streaming_io  run_time_configurable_transform_length=off  phase_factor_width=16  scaling_options=unscaled  rounding_modes=truncation  aclken=off  aresetn=off  output_ordering=natural_order  cyclic_prefix_insertion=off  throttle_scheme=nonrealtime  xk_index=on  ovflo=off  trim_axipin_name=on  memory_options_data=block_ram  memory_options_phase_factors=block_ram  number_of_stages_using_block_ram_for_data_and_phase_factors=2  memory_options_reorder=block_ram  memory_options_hybrid=off  complex_mult_type=use_mults_resources  butterfly_type=use_luts  simulation_type=hybrid_sim  simulation_model=sysgen:xfftv9_cmodel  data_path_portlist={ 's_axis_data_tdata', 'm_axis_data_tdata', 'm_axis_status_tdata', 'event_fft_overflow' }  channels=1  input_ordering=natural_order  input_width=16  ip_name=Fast Fourier Transform  ip_version=9.1  dsptool_ready=true  ipcore_usecache=true  ipcore_useipmodelcache=true  wrapper_available=true  port_translation_map={ 'aclken' => 'en', 'aresetn' => 'rst'}  data_format=fixed_point  block_type=xfft_v9_1
  NCO : Subsystem  mask(Numerically Controller Oscillator (NCO)){fs=8000, n=10, L=16}
      mask prompts: fs "Sampling frequency"; n "Lookup table address size"; L "Precision of output (total bits, 2 of which integer)"
      mask help: Parameteristable NCO producing sine and cosine outputs.
      mask init:
      | N = 2^n;    % size (depth) of lookup table
      | 
      | i = ceil(log2(ceil(N/fs)))+1;   % calculate integer and fractional bits
      | b = 10;                         % required for constant (in conversion to step size)
  Product : xbsIndex_r4/Product  complex_multiplier=on  optimizegoal=Performance  simulation_type=fast_sim  simulation_model=sysgen:product_macro  block_type=product_macro
  Product1 : xbsIndex_r4/Product  complex_multiplier=on  optimizegoal=Performance  simulation_type=fast_sim  simulation_model=sysgen:product_macro  block_type=product_macro
  Product2 : xbsIndex_r4/Product  complex_multiplier=on  optimizegoal=Performance  simulation_type=fast_sim  simulation_model=sysgen:product_macro  block_type=product_macro
  Scaled Mag Squared FFT : Subsystem
  Corrected_I : Outport
  Corrected_Q : Outport  Port=2
  tvalid_out : Outport  Port=3
  wires:
  I_samples/1 -> Product2/1, Product/1, Product/3
  Q_samples/1 -> Product/4, Product2/2, Product/2
  Product/1 -> Convert/1
  Product/2 -> Convert1/1
  Product1/1 -> Convert2/1
  Product1/2 -> Convert3/1
  Convert/1 -> Product1/3, Product1/1
  Convert1/1 -> Product1/4, Product1/2
  Convert2/1 -> FFT/4
  Convert3/1 -> FFT/3
  Delay1/1 -> FFT/5, FFT/6
  Constant2/1 -> FFT/7
  Constant4/1 -> FFT/2
  Constant3/1 -> FFT/1
  FFT/3 -> Scaled Mag Squared FFT/1(Im)
  FFT/4 -> Scaled Mag Squared FFT/2(Re)
  FFT/5 -> Scaled Mag Squared FFT/3(FFT_Index)
  FFT/6 -> Scaled Mag Squared FFT/4(Valid)
  NCO/1(cos) -> Product2/3
  NCO/2(sin) -> Product2/4
  Determine Frequency Correction Term/1(Freq_correction) -> NCO/1(freq_correction)
  Scaled Mag Squared FFT/1(Mag_Sq_FFT) -> Determine Frequency Correction Term/1(Mag_Sq_FFT)
  Scaled Mag Squared FFT/2(FFT_index_del) -> Determine Frequency Correction Term/2(FFT_index)
  Scaled Mag Squared FFT/3(Valid_del) -> Determine Frequency Correction Term/3(Valid)
  Determine Frequency Correction Term/2(Valid_out) -> NCO/2(en)
  Product2/1 -> Convert4/1
  Product2/2 -> Convert5/1
  Convert4/1 -> Corrected_I/1
  Convert5/1 -> Corrected_Q/1
  tvalid_in/1 -> Delay/1
  Delay/1 -> Delay1/1
  NCO/3(tvalid) -> Delay2/1
  Delay2/1 -> tvalid_out/1

== system AXI_QPSK_Rx/Subsystem/Data Inspector ==
  symbol_i_data : Inport
  symbol_i_valid : Inport  Port=2
  symbol_q_data : Inport  Port=3
  reset : Inport  Port=4
  packet_size : Inport  Port=5
  transfer : Inport  Port=6
  auto_restart : Inport  Port=7
  tready_in : Inport  Port=8
  M_AXIS_SYMBOL_CTRL : Subsystem
  tdata_out : Outport
  tvalid_out : Outport  Port=2
  tlast_out : Outport  Port=3
  wires:
  symbol_i_data/1 -> M_AXIS_SYMBOL_CTRL/1(i_data)
  symbol_i_valid/1 -> M_AXIS_SYMBOL_CTRL/2(tvalid_in)
  symbol_q_data/1 -> M_AXIS_SYMBOL_CTRL/3(q_data)
  reset/1 -> M_AXIS_SYMBOL_CTRL/4(reset)
  packet_size/1 -> M_AXIS_SYMBOL_CTRL/5(packet_size)
  tready_in/1 -> M_AXIS_SYMBOL_CTRL/6(tready_in)
  M_AXIS_SYMBOL_CTRL/1(tdata_out) -> tdata_out/1
  M_AXIS_SYMBOL_CTRL/2(tvalid_out) -> tvalid_out/1
  M_AXIS_SYMBOL_CTRL/3(tlast_out) -> tlast_out/1
  transfer/1 -> M_AXIS_SYMBOL_CTRL/7(transfer)
  auto_restart/1 -> M_AXIS_SYMBOL_CTRL/8(auto_restart)

== system AXI_QPSK_Rx/Subsystem/Data Inspector Decimation ==
  symbol_i_data : Inport
  symbol_i_valid : Inport  Port=2
  symbol_q_data : Inport  Port=3
  reset : Inport  Port=4
  packet_size : Inport  Port=5
  transfer : Inport  Port=6
  auto_restart : Inport  Port=7
  tready_in : Inport  Port=8
  M_AXIS_SYMBOL_CTRL : Subsystem
  tdata_out : Outport
  tvalid_out : Outport  Port=2
  tlast_out : Outport  Port=3
  wires:
  symbol_i_data/1 -> M_AXIS_SYMBOL_CTRL/1(i_data)
  symbol_i_valid/1 -> M_AXIS_SYMBOL_CTRL/2(tvalid_in)
  symbol_q_data/1 -> M_AXIS_SYMBOL_CTRL/3(q_data)
  reset/1 -> M_AXIS_SYMBOL_CTRL/4(reset)
  packet_size/1 -> M_AXIS_SYMBOL_CTRL/5(packet_size)
  tready_in/1 -> M_AXIS_SYMBOL_CTRL/6(tready_in)
  M_AXIS_SYMBOL_CTRL/1(tdata_out) -> tdata_out/1
  M_AXIS_SYMBOL_CTRL/2(tvalid_out) -> tvalid_out/1
  M_AXIS_SYMBOL_CTRL/3(tlast_out) -> tlast_out/1
  transfer/1 -> M_AXIS_SYMBOL_CTRL/7(transfer)
  auto_restart/1 -> M_AXIS_SYMBOL_CTRL/8(auto_restart)

== system AXI_QPSK_Rx/Subsystem/Data Inspector Freq Sync ==
  symbol_i_data : Inport
  symbol_i_valid : Inport  Port=2
  symbol_q_data : Inport  Port=3
  reset : Inport  Port=4
  packet_size : Inport  Port=5
  transfer : Inport  Port=6
  auto_restart : Inport  Port=7
  tready_in : Inport  Port=8
  M_AXIS_SYMBOL_CTRL : Subsystem
  tdata_out : Outport
  tvalid_out : Outport  Port=2
  tlast_out : Outport  Port=3
  wires:
  auto_restart/1 -> M_AXIS_SYMBOL_CTRL/8(auto_restart)
  transfer/1 -> M_AXIS_SYMBOL_CTRL/7(transfer)
  M_AXIS_SYMBOL_CTRL/3(tlast_out) -> tlast_out/1
  M_AXIS_SYMBOL_CTRL/2(tvalid_out) -> tvalid_out/1
  M_AXIS_SYMBOL_CTRL/1(tdata_out) -> tdata_out/1
  tready_in/1 -> M_AXIS_SYMBOL_CTRL/6(tready_in)
  packet_size/1 -> M_AXIS_SYMBOL_CTRL/5(packet_size)
  reset/1 -> M_AXIS_SYMBOL_CTRL/4(reset)
  symbol_q_data/1 -> M_AXIS_SYMBOL_CTRL/3(q_data)
  symbol_i_valid/1 -> M_AXIS_SYMBOL_CTRL/2(tvalid_in)
  symbol_i_data/1 -> M_AXIS_SYMBOL_CTRL/1(i_data)

== system AXI_QPSK_Rx/Subsystem/Data Inspector RRC ==
  symbol_i_data : Inport
  symbol_i_valid : Inport  Port=2
  symbol_q_data : Inport  Port=3
  reset : Inport  Port=4
  packet_size : Inport  Port=5
  transfer : Inport  Port=6
  auto_restart : Inport  Port=7
  tready_in : Inport  Port=8
  M_AXIS_SYMBOL_CTRL : Subsystem
  tdata_out : Outport
  tvalid_out : Outport  Port=2
  tlast_out : Outport  Port=3
  wires:
  auto_restart/1 -> M_AXIS_SYMBOL_CTRL/8(auto_restart)
  transfer/1 -> M_AXIS_SYMBOL_CTRL/7(transfer)
  M_AXIS_SYMBOL_CTRL/3(tlast_out) -> tlast_out/1
  M_AXIS_SYMBOL_CTRL/2(tvalid_out) -> tvalid_out/1
  M_AXIS_SYMBOL_CTRL/1(tdata_out) -> tdata_out/1
  tready_in/1 -> M_AXIS_SYMBOL_CTRL/6(tready_in)
  packet_size/1 -> M_AXIS_SYMBOL_CTRL/5(packet_size)
  reset/1 -> M_AXIS_SYMBOL_CTRL/4(reset)
  symbol_q_data/1 -> M_AXIS_SYMBOL_CTRL/3(q_data)
  symbol_i_valid/1 -> M_AXIS_SYMBOL_CTRL/2(tvalid_in)
  symbol_i_data/1 -> M_AXIS_SYMBOL_CTRL/1(i_data)
